simulink library "cjt_library_controllers"  (Simulink 9.0)
settings: Solver=ode45  StartTime=0.0  StopTime=10.0  RelTol=1e-3  EnableMultiTasking=on
values from neighbouring files (symbols this model uses):
  N = this.jointModel.n    [dataSheetGenerator.m]
undefined symbols (not defined in the file or in its folder): Cc, D, DiscIntNeverNeededParam, dob_switch, jointObj, K_lqr, kest
undefined symbols (not defined in the file): My_joint
libraries: cstblocks x6, cjt_library_observers x2
settings Model: Creator=wesley  LastModifiedBy=J�rn

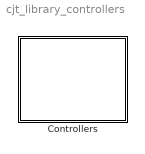
== system cjt_library_controllers ==
  Controllers : Subsystem

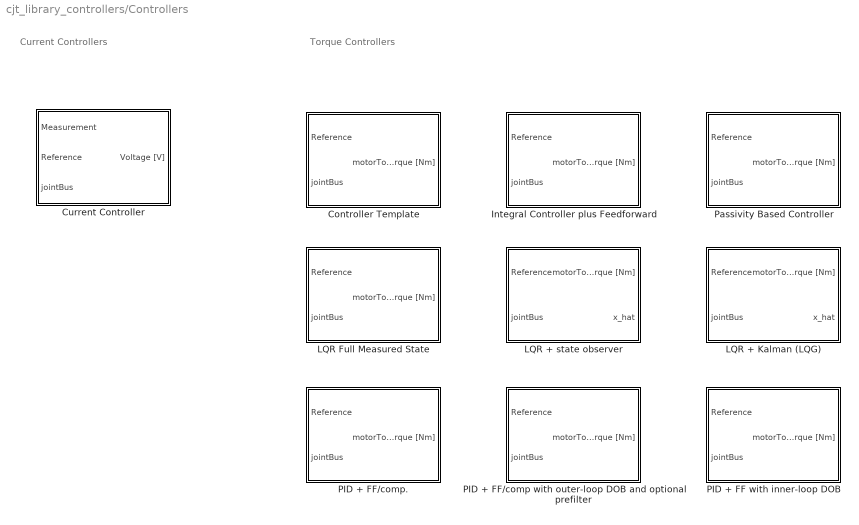
== system cjt_library_controllers/Controllers ==
  note: Torque Controllers
  note: Current Controllers
  Controller Template : Subsystem  mask(CJT Controller Template){jointObj=jointObj}
      mask prompts: jointObj "Joint Object"
      mask help:
      | This is a template block. If you have a controller that you wish to contribute to this library, this block here  represents your interface.
      |
      | Here are the steps to contribute your controller using this template:
      |
      | 1. Copy this block into your development. Disable and break its link to this library. You now have a copy of the interface in your model that is disconnected from the library.
      |
      | 2. Implement your controller within this block. The controller should use no hardcoded values. Wherever you can, access the properties of a CJT joint object. The joint object should be passed to the block through the mask as first parameter (e.g. jointObj).
      |
      | 3. Complete the block mask, so the user can specify all block properties programatically or manually through the mask.
      |
      | 4. Make an example:
      | a) Clean your development model up and convert it into a minimum example that demonstrates the use of your block.
      | b) Create an m-script that configures the required joint object and simulation parameters, runs the model.and displays some results. See existing examples and copy their format.
      | c) Write the documentation of your block.
      |
      | 5. Write a unit test. Look into the unit test directory and open the unit test file for this library. Add a test for your block. A good point to start is your example. Make the test pass.
      |
      | 6. Submit your contribution!
      |
      | Thanks a lot!
      |
      | 7.
      mask init:
      | % Do all the controller related computations here.
      | % Compute gains etc.
      | 
      | % E.g. get linear dynamics matrices first...
      | [A, B, C, I, D, K] = jointObj.getDynamicsMatrices();
      | 
      | % YOUR CODE HERE
      mask Help:
      | This is a template block. If you have a controller that you wish to contribute to this library, this block here  represents your interface.
      | 
      | Here are the steps to contribute your controller using this template:
      | 
      | 1. Copy this block into your development. Disable and break its link to this library. You now have a copy of the interface in your model that is disconnected from the library.
      | 
      | 2. Implement your controller within this block. The controller should use no hardcoded values. Wherever you can, access the properties of a CJT joint object. The joint object should be passed to the block through the mask as first parameter (e.g. jointObj).
      | 
      | 3. Complete the block mask, so the user can specify all block properties programatically or manually through the mask.
      | 
      | 4. Make an example:
      | a) Clean your development model up and convert it into a minimum example that demonstrates the use of your block.
      | b) Create an m-script that configures the required joint object and simulation parameters, runs the model.and displays some results. See existing examples and copy their format.
      | c) Write the documentation of your block.
      | 
      | 5. Write a unit test. Look into the unit test directory and open the unit test file for this library. Add a test for your block. A good point to start is your example. Make the test pass.
      | 
      | 6. Submit your contribution!
      | 
      | Thanks a lot!
  Current Controller : Subsystem  mask(CJT Torque Controller){jointObj=My_joint, P_Gain=1, I_Gain=0.05, ff_chk=on, bemf_chk=on}
      mask prompts: jointObj "Joint Object"; P_Gain "Proportional Gain"; I_Gain "Integral Gain"; ff_chk "Feedforward Action"; bemf_chk "Back EMF Compensation"
      mask help:
      | The block implements a PI current controller augmented by a voltage feedforward term and a back-EMF compensation based on motor velocity readings.
      |
      | This block serves in combination with an electrical subsystem block.
      |
      | Click >Help< for details on the parameters.
      mask init:
      | ff_enable = 0;
      | if ff_chk
      |     ff_enable = 1.0;
      | end
      | 
      | bemf_enable = 0;
      | if bemf_chk
      |     bemf_enable = 1.0;
      | end
      mask Help:
      | The block implements a PI current controller augmented by a voltage feedforward term and a back-EMF compensation based on motor velocity readings.
      | 
      | This block serves in combination with an electrical subsystem block.
      | 
      | <b>Mask parameters:</b>
      | 
      | Joint Object:  The class name of the CJT joint class name or the variable representing an instance of a CJT joint class, describing the
      | 
      | Proportional Gain: PI controller P-gain
      | Integral Gain: PI controller I-gain
      | 
      | Feedforward Action: check, if feedforward action is desired.
      | Back EMF Compensation : check, if back EMF compensation shall be active .
  Integral Controller plus Feedforward : Subsystem  mask(CJT Torque Controller){jointObj=jointObj, I_Gain=10}
      mask prompts: jointObj "Joint Object"; I_Gain "Integral gain K_I"
      mask help:
      | The block implements a torque controller comprised of a feedforward term complemented by an integral action with gain K_I to compensate for disturbances.
      |
      | Click >Help< for further documentation.
      mask Help:
      | The block implements a torque controller comprised of a feedforward term complemented by an integral action to compensate for disturbances. This type of controller has been used and discussed as lag-type control design in comparison to a pure feedforward action as well as a Proportional-Derivative control action in [1].
      | 
      | <b>Mask parameters:</b>
      | 
      | Joint Object:  The class name of the CJT joint class name or the variable representing an instance of a CJT joint class, describing the
      | 
      | K<sub>I</sub>: Integral gain
      | 
      | According to [1] the controller reduces disturbances up to a frequency <i>f = K<sub>I</sub>  / ( 2 PI ). </i>
      | 
      | <b>References:</b>
      | [1] D. Vischer and O. Khatib, â€œDesign and development of high-performance torque-controlled joints,â€ Robotics and Automation, IEEE Transactions on, vol. 11, no. 4, pp. 537â€“544, 1995.
      | [2] M. C. Readman, Flexible Joint Robots. CRC press, 1994.
  LQR + Kalman (LQG) : Subsystem  mask{jointObj=jointObj, outputIdx=7, Q=diag([0 0 1000 0 0 0]), R=5e-6, var_u=0.12^2, var_y=1.8e-10}
      mask prompts: jointObj "Joint Object (fixed output model)"; outputIdx "Measured output"; Q "State weighing matrix Q"; R "Input weighing matrix R"; var_u "Input noise variance"; var_y "Measurement noise variance"
      mask init:
      | % Get linear dynamics matrices
      | [A, B, C, D] = jointObj.getDynamicsMatrices();
      | 
      | % Parameters
      | N_outputs       = size(C,1);
      | 
      | % Get LQR gain and Kalman observer
      | [K_lqr, N]  	= getLQR(jointObj, outputIdx, Q, R);
      | [kest, L, Cc]	= getKalman(jointObj, outputIdx, var_u, var_y);
      | 
      | % Indexes of output states
      | kest_stateIdx   = kest.OutputGroup.StateEstimate;
      | 
      | % Discretize using Tustin transform
      | kest_tust       = c2d(kest, jointObj.Ts, 'tustin');
  LQR + state observer : Subsystem  mask{jointObj=jointObj, outputIdx=7, Q=diag([0 0 1000 0 0 0]), R=5e-6, place_gain=4}
      mask prompts: jointObj "Joint Object"; outputIdx "Measured output"; Q "State weighing matrix Q"; R "Input weighing matrix R"; place_gain "Pole placement gain"
      mask init:
      | % Get linear dynamics matrices
      | [A, B, C, D] = jointObj.getDynamicsMatrices();
      | 
      | % Parameters
      | N_outputs = size(C,1);
      | 
      | % Get LQR gain and state observer
      | [K_lqr, N]          = getLQR(jointObj, outputIdx, Q, R);
      | [sys_hat, L, Cc]	= getObserver(jointObj, outputIdx, place_gain, Q, R);
      | 
      | % Discretize using Tustin transform
      | sys_hat_tust = c2d(sys_hat, jointObj.Ts, 'tustin');
  LQR Full Measured State : Subsystem  mask{jointObj=My_joint, outputIdx=7, Q=diag([0 0 1000 0 0 0]), R=5e-6}
      mask prompts: jointObj "Joint Object"; outputIdx "Measured output"; Q "State weighing matrix Q"; R "Input weighing matrix R"
      mask init:
      | % Get linear dynamics matrices
      | [A, B, C, D] = jointObj.getDynamicsMatrices();
      | 
      | % Get LQR gain and premultiplication matrix N
      | [K_lqr, N]          = getLQR(jointObj, outputIdx, Q, R);
      | 
      | % Get selector to obtain full state from outputs y
      | % This makes use of the fact that the first 6 outputs are the states
      | outputToStates      = C(1:6,:)';
  PID + FF with inner-loop DOB : Subsystem  mask(PID + FF with inner-loop DOB){jointObj=jointObj, Kp=1, Ki=0, Kd=0, N=2*pi*200, ff_comp_switch=Feed-forward, DOB_enabled=on, f_c=100, measIdx=[7]}
      mask prompts: jointObj "Joint Object"; Kp "Proportional gain Kp"; Ki "Integral gain Ki"; Kd "Derivative gain Kd"; N "Filter coefficient N"; ff_comp_switch "Spring force rejection"; DOB_enabled "DOB enabled"; f_c "DOB cut-off frequency [Hz]"; measIdx "Measurement index"
      mask help:
      | This block implements a PID torque controller with optional feed-forward or compensation term, supplemented with an inner-loop DOB.
      |
      | Click >Help< for further documentation.
      mask init:
      | % Get linear dynamics matrices
      | [A, B, C, D, I, R, K] = jointObj.getDynamicsMatrices();
      mask Help:
      | This block implements a PID torque controller with optional feed-forward or compensation term, supplemented with an inner-loop DOB. The DOB is based on the nominal open-loop plant dynamics.
      | 
      | <b>Mask parameters:</b>
      | 
      | Joint Object: The class name of the CJT joint class name or the variable representing an instance of a CJT joint class.
      | K<sub>P</sub>, K<sub>I</sub>, K<sub>D</sub>: Proportional, derivative, and integral gain, respectively.
      | N: Derivative low-pass filter coefficient
      | DOB cutoff frequency: Cut-off frequency computed for the low-pass filter that must be used to make the inverse transfer function realisible.
      | Measurement index: Measured plant output that should be used for the DOB.
      | 
      | 
      | <b>References:</b>
      | 
      | H. S. Lee and M. Tomizuka, "Robust motion controller design for high-accuracy positioning systems". In IEEE Transactions on Industrial Electronics, vol. 43, no. 1, pp. 48--55, 1996.
      | 
      | W. Roozing, J. Malzahn, D. G. Caldwell, and N. G. Tsagarakis, "Comparison of open-loop and closed-loop disturbance observers for series elastic actuators". In Intelligent Robots and Systems (IROS), 2016 IEEE/RSJ International Conference on, 2016, pp. 3842--3847.
      | 
      | M. C. Readman, Flexible Joint Robots. CRC press, 1994.
      mask TypeOptions ff_comp_switch: Compensation | Feed-forward | Off
      mask Callback DOB_enabled:
      | % Toggle all DOB fields
      | fields = {  'f_c', ...
      |             'measIdx'
      |          };
      | toggleMaskFields(gcbh, 'DOB_enabled', fields, 'on');
      mask DialogControl Container3 Prompt: Controller
      mask DialogControl ParameterGroupVar Prompt: DOB parameters
  PID + FF/comp with outer-loop DOB and optional prefilter : Subsystem  mask(PID + FF/comp with outer-loop DOB and optional prefilter){jointObj=jointObj, Kp=0.1, Ki=0, Kd=0.001, N=2*pi*200, ff_comp_switch=Feed-forward, DOB_enable_switch=On, premult_enable_switch=Off, loadData=off, modelFname=DOB_results.mat, f_c_FF=50, f_c_DOB=80}
      mask prompts: jointObj "Joint Object"; Kp "Proportional gain Kp"; Ki "Integral gain Ki"; Kd "Derivative gain Kd"; N "Derivative filter coefficient N"; ff_comp_switch "Spring force rejection"; DOB_enable_switch "DOB"; premult_enable_switch "Premultiplication"; loadData "Load model/filters from file (see getLinearDOB_fromData)"; modelFname "Model/filters file (.mat)"; f_c_FF "Premultiplication (model inversion) cutoff frequency [Hz]"; f_c_DOB "DOB cutoff frequency [Hz]"
      mask help:
      | This block implements a PID torque controller with optional feed-forward or compensation term, supplemented with an outer-loop DOB and optional prefilter.
      |
      | Click >Help< for further documentation.
      mask init:
      | mask_PID_FFComp_OuterLoopDOB
      mask Help:
      | This block implements a PID torque controller with optional feed-forward or compensation term, supplemented with an outer-loop DOB and optional prefilter. The DOB is based on a nominal model of the closed control loop. Multiplication by the prefilter simply means taking the inverse of the closed-loop as premultiplication, with a low-pass filter, very similar to a classical lead filter.
      | 
      | <b>Mask parameters:</b>
      | 
      | Joint Object: The class name of the CJT joint class name or the variable representing an instance of a CJT joint class.
      | K<sub>P</sub>, K<sub>I</sub>, K<sub>D</sub>: Proportional, derivative, and integral gain, respectively.
      | N: Derivative low-pass filter coefficient
      | Models/filters file: Instead of analytical computation from the given joint model, a DOB model can be loaded from file, that is e.g. computed from experimental data.
      | Premultiplication and DOB cutoff frequency: Cut-off frequency computed for the low-pass filters that must be used to make the inverse transfer functions realisible.
      | 
      | 
      | <b>References:</b>
      | 
      | M. C. Readman, Flexible Joint Robots. CRC press, 1994.
      | 
      | K. Kong, J. Bae, and M. Tomizuka, "Control of Rotary Series Elastic Actuator for Ideal Force-Mode Actuation in Human-Robot Interaction Applications". In: IEEE/ASME Transactions on Mechatronics, vol. 14, no. 1, pp. 105--118, Feb. 2009.
      | 
      | N. Paine, S. Oh, and L. Sentis, "Design and Control Considerations for High-Performance Series Elastic Actuators". In: IEEE/ASME Transactions on Mechatronics, vol. 19, no. 3, pp. 1080--1091, Jun. 2014.
      | 
      | N. Paine, J. S. Mehling, J. Holley, N. A. Radford, G. Johnson, C.-L. Fok, and L. Sentis, "Actuator Control for the NASA-JSC Valkyrie Humanoid Robot: A Decoupled Dynamics Approach for Torque Control of Series Elastic Robots: Actuator Control for the NASA-JSC Valkyrie Humanoid Robot". In: Journal of Field Robotics, vol. 32, no. 3, pp. 378--396, May 2015.
      | 
      | J. S. Mehling, J. Holley, and M. K. O'Malley, "Leveraging disturbance observer based torque control for improved impedance rendering with series elastic actuators". In: IEEE/RSJ International Conference on Intelligent Robots and Systems (IROS), 2015, pp. 1646--1651.
      | 
      | W. Roozing, J. Malzahn, D. G. Caldwell, and N. G. Tsagarakis, "Comparison of open-loop and closed-loop disturbance observers for series elastic actuators". In:  IEEE/RSJ International Conference on Intelligent Robots and Systems (IROS), 2016, pp. 3842--3847.
      mask TypeOptions ff_comp_switch: Compensation | Feed-forward | Off
      mask TypeOptions DOB_enable_switch: Off | On
      mask Callback DOB_enable_switch:
      | % Toggle all DOB fields
      | fields = {  'premult_enable_switch', ...
      |             'loadData', ...
      |             'modelFname', ...
      |             'id_Np', ...
      |             'id_Nz', ...
      |             'f_c_FF', ...
      |             'f_c_DOB', ...
      |          };
      | toggleMaskFields(gcbh, 'DOB_enable_switch', fields, 'on');
      | 
      | % File load or model generation
      | if (strcmpi(get(gcbh, 'DOB_enable_switch'), 'on'))
      |     toggleMaskFields(gcbh, 'loadData', 'modelFname', 'on');
      |     toggleMaskFields(gcbh, 'loadData', {'f_c_FF', 'f_c_DOB'}, 'off');
      | end
      mask TypeOptions premult_enable_switch: Off | On
      mask Callback loadData:
      | if (strcmpi(get(gcbh, 'DOB_enable_switch'), 'on'))
      |     toggleMaskFields(gcbh, 'loadData', 'modelFname', 'on');
      |     toggleMaskFields(gcbh, 'loadData', {'button_build_DOB', 'f_c', 'id_Np', 'id_Nz', 'f_c_FF', 'f_c_DOB'}, 'off');
      | end
      mask DialogControl Container2 Prompt: Controller
      mask DialogControl DOB_container Prompt: DOB and premultiplication
      mask DialogControl DOB_analytical_container Prompt: Analytical DOB
  PID + FF/comp. : Subsystem  mask(PID + FF/comp.){jointObj=jointObj, Kp=2, Ki=0, Kd=0.01, N=2*pi*200, ff_comp_switch=Feed-forward}
      mask prompts: jointObj "Joint Object"; Kp "Proportional gain Kp"; Ki "Integral gain Ki"; Kd "Derivative gain Kd"; N "Filter coefficient N"; ff_comp_switch "Feed-forward/compensation"
      mask help:
      | This block implements a PID torque controller with optional feed-forward or compensation term.
      |
      | Click >Help< for further documentation.
      mask init:
      | % Get linear dynamics matrices
      | [A, B, C, D, I, R, K] = jointObj.getDynamicsMatrices();
      mask Help:
      | This block implements a PID torque controller with optional feed-forward or compensation term.
      | 
      | <b>Mask parameters:</b>
      | 
      | Joint Object: The class name of the CJT joint class name or the variable representing an instance of a CJT joint class.
      | K<sub>P</sub>, K<sub>I</sub>, K<sub>D</sub>: Proportional, derivative, and integral gain, respectively.
      | N: Derivative low-pass filter coefficient
      | 
      | 
      | <b>References:</b>
      | 
      | M. C. Readman, Flexible Joint Robots. CRC press, 1994.
      mask TypeOptions ff_comp_switch: Compensation | Feed-forward | Off
  Passivity Based Controller : Subsystem  mask(Passivity Based Torque Controller with Optional Generalized Momentum Based Disturbance Observer){jointObj=jointObj, BBinv=4, Ds=25, isDOBActive=on, L=2*pi*60}
      mask prompts: jointObj "Joint Object"; BBinv "Inertia Scaling"; Ds "Damping"; isDOBActive "DOB Active"; L "Gain L"
      mask help:
      | This block implements a passivity based torque controller. It has two positive valued parameters. The first parameter is a downscaling factor for the apparent inertia. The second parameter adds damping in proportion to the spring deflection rate. The controller relies on the knowledge of the joint intrinsic stiffness and damping provided through the joint class.
      |
      | The controller can be augmented by a generalized momentum based disturbance observer. The observer outputs a low-pass filtered version of the actual disturbance and  introduces one additional parameter. The parameter is the cut-off frequency of the low-pass filter in radians/s. The observer relies on the knowledge of the joint inertia provided through the joint class.
      |
      | Click >Help< for further documentation.
      mask init:
      | mask_Passivity_Based_Control
      mask Help:
      | This block implements the passivity based torque controller presented by Alin Albu-Schäffer, Christian Ott  and Gerd Hirzinger (2007).
      | It has two positive valued parameters. The first parameter is a downscaling factor for the apparent inertia. The second parameter adds damping in proportion to the spring deflection rate. The controller relies on the knowledge of the joint intrinsic stiffness and damping provided through the joint object.
      | 
      | The controller can be augmented by a generalized momentum based disturbance observer as described by Luc Le Tien  et al (2008).. The observer outputs a low-pass filtered version of the actual disturbance and  introduces one additional parameter. The parameter is the cut-off frequency of the low-pass filter in radians/s. The observer relies on the knowledge of the joint inertia provided through the joint class.
      | 
      | 
      | <b>Mask parameters:</b>
      | 
      | Joint Object: The class name of the CJT joint class name or the variable representing an instance of a CJT joint class.
      | Inertia Scaling: This parameter is a proportional gain on the torque error. It acts as an inertia downscaling factor. The apparent joint inertia proportionally increases for values < 0 and decreases for parameter values > 1
      | Damping: This parameter is a derivative gain on the joint deflection measurement. It adds damping in direct proportion to the joint deflection rate.
      | DOB Active: if checked, the controller is augmented by the generalized momentum based disturbance observer.
      | Gain L: Disturbance observer gain that essentially is the cut-off frequency of a low-pass filter for the actual real disturbance given in radians/s.
      | 
      | 
      | <b>References:</b>
      | Albu-Schäffer, Alin, Christian Ott, and Gerd Hirzinger. "A unified passivity-based control framework for position, torque and impedance control of flexible joint robots." The international journal of robotics research 26.1 (2007): 23-39.
      | 
      | Le Tien, Luc, et al. "Friction observer and compensation for control of robots with joint torque measurement." Intelligent Robots and Systems, 2008. IROS 2008. IEEE/RSJ International Conference on. IEEE, 2008.
      mask Callback isDOBActive:
      | maskObj = Simulink.Mask.get(gcb);
      | 
      | maskObj.Parameters(5).Enabled = maskObj.Parameters(4).Value;
      mask DialogControl Controller_container Prompt: Controller
      mask DialogControl DOB_container Prompt: Disturbance Observer (DOB)

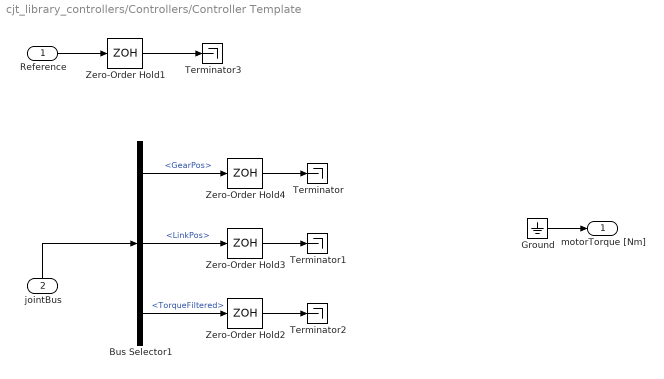
== system cjt_library_controllers/Controllers/Controller Template ==
  Reference : Inport
  jointBus : Inport  Port=2
  Bus Selector1 : BusSelector  OutputSignals=GearPos,LinkPos,TorqueFiltered
  Ground : Ground
  Terminator{,1..3} (4 alike) : Terminator
  Zero-Order Hold{1..4} (4 alike) : ZeroOrderHold  SampleTime=jointObj.Ts
  motorTorque [Nm] : Outport
  wires:
  jointBus/1 -> Bus Selector1/1
  Bus Selector1/1 -> Zero-Order Hold4/1  "<GearPos>"
  Bus Selector1/2 -> Zero-Order Hold3/1  "<LinkPos>"
  Bus Selector1/3 -> Zero-Order Hold2/1  "<TorqueFiltered>"
  Reference/1 -> Zero-Order Hold1/1
  Ground/1 -> motorTorque [Nm]/1
  Zero-Order Hold1/1 -> Terminator3/1
  Zero-Order Hold2/1 -> Terminator2/1
  Zero-Order Hold3/1 -> Terminator1/1
  Zero-Order Hold4/1 -> Terminator/1

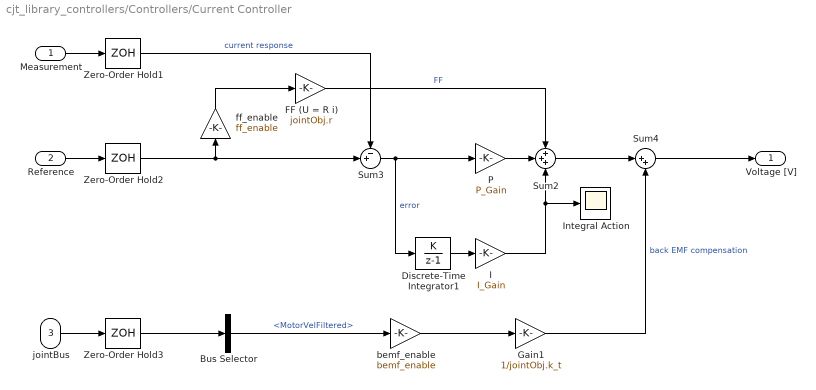
== system cjt_library_controllers/Controllers/Current Controller ==
  Measurement : Inport
  Reference : Inport  Port=2
  jointBus : Inport  Port=3
  Bus Selector : BusSelector  OutputSignals=MotorVelFiltered
  Discrete-Time Integrator1 : DiscreteIntegrator  IntegratorMethod=Accumulation: Forward Euler  SampleTime=jointObj.Ts_elec  ICPrevOutput=DiscIntNeverNeededParam  ICPrevScaledInput=DiscIntNeverNeededParam
  FF (U = R i) : Gain  Gain=jointObj.r
  Gain1 : Gain  Gain=1/jointObj.k_t
  I : Gain  Gain=I_Gain
  Integral Action : Scope
  P : Gain  Gain=P_Gain
  Sum2 : Sum  Inputs=+++
  Sum3 : Sum  Inputs=-+|
  Sum4 : Sum  Inputs=|++
  Zero-Order Hold1 : ZeroOrderHold  SampleTime=jointObj.Ts_elec
  Zero-Order Hold2 : ZeroOrderHold  SampleTime=jointObj.Ts_elec
  Zero-Order Hold3 : ZeroOrderHold  SampleTime=jointObj.Ts_elec
  bemf_enable : Gain  Gain=bemf_enable
  ff_enable : Gain  Gain=ff_enable
  Voltage [V] : Outport
  wires:
  Reference/1 -> Zero-Order Hold2/1
  jointBus/1 -> Zero-Order Hold3/1
  FF (U = R i)/1 -> Sum2/1  "FF"
  I/1 -> Sum2/3, Integral Action/1
  Discrete-Time Integrator1/1 -> I/1
  Sum2/1 -> Sum4/1
  Measurement/1 -> Zero-Order Hold1/1
  Gain1/1 -> Sum4/2  "back EMF compensation"
  P/1 -> Sum2/2
  Sum3/1 -> Discrete-Time Integrator1/1, P/1  "error"
  Bus Selector/1 -> bemf_enable/1  "<MotorVelFiltered>"
  ff_enable/1 -> FF (U = R i)/1
  bemf_enable/1 -> Gain1/1
  Zero-Order Hold1/1 -> Sum3/1  "current response"
  Zero-Order Hold2/1 -> ff_enable/1, Sum3/2
  Zero-Order Hold3/1 -> Bus Selector/1
  Sum4/1 -> Voltage [V]/1

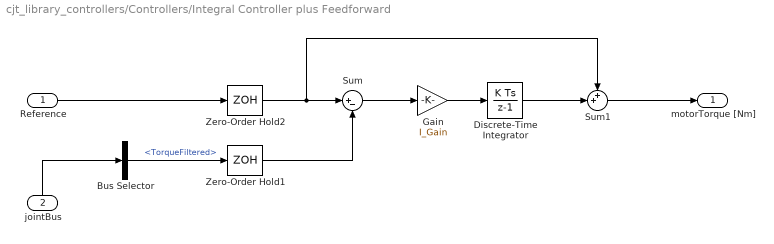
== system cjt_library_controllers/Controllers/Integral Controller plus Feedforward ==
  Reference : Inport
  jointBus : Inport  Port=2
  Bus Selector : BusSelector  OutputSignals=TorqueFiltered
  Discrete-Time Integrator : DiscreteIntegrator  InitialConditionSetting=State (most efficient)  SampleTime=jointObj.Ts  ICPrevOutput=DiscIntNeverNeededParam  ICPrevScaledInput=DiscIntNeverNeededParam
  Gain : Gain  Gain=I_Gain
  Sum : Sum  Inputs=|+-
  Sum1 : Sum  Inputs=++|
  Zero-Order Hold1 : ZeroOrderHold  SampleTime=jointObj.Ts
  Zero-Order Hold2 : ZeroOrderHold  SampleTime=jointObj.Ts
  motorTorque [Nm] : Outport
  wires:
  jointBus/1 -> Bus Selector/1
  Reference/1 -> Zero-Order Hold2/1
  Bus Selector/1 -> Zero-Order Hold1/1  "<TorqueFiltered>"
  Sum/1 -> Gain/1
  Gain/1 -> Discrete-Time Integrator/1
  Discrete-Time Integrator/1 -> Sum1/2
  Sum1/1 -> motorTorque [Nm]/1
  Zero-Order Hold1/1 -> Sum/2
  Zero-Order Hold2/1 -> Sum/1, Sum1/1

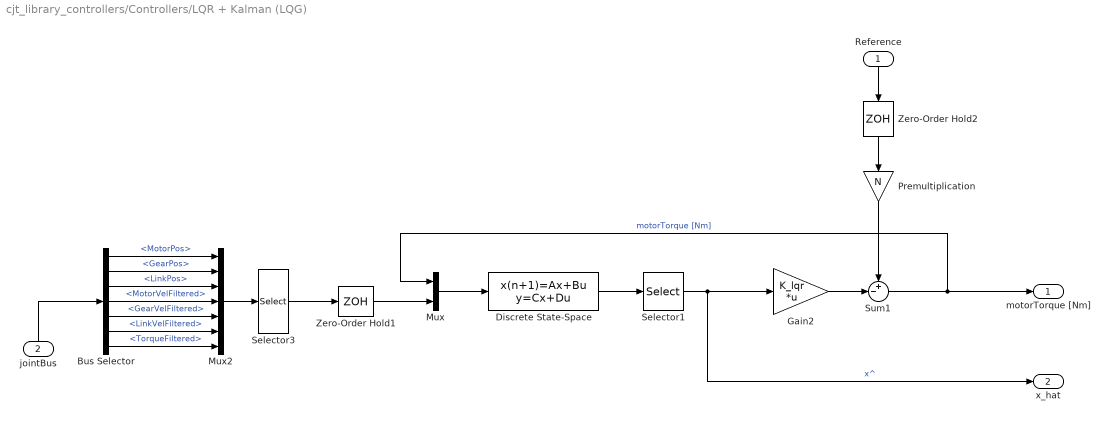
== system cjt_library_controllers/Controllers/LQR + Kalman (LQG) ==
  Reference : Inport
  jointBus : Inport  Port=2
  Bus Selector : BusSelector  OutputSignals=MotorPos,GearPos,LinkPos,MotorVelFiltered,GearVelFiltered,LinkVelFiltered,TorqueFiltered
  Discrete State-Space : DiscreteStateSpace  A=kest_tust.a  B=kest_tust.b  C=kest_tust.c  D=kest_tust.d  SampleTime=jointObj.Ts
  Gain2 : Gain  Gain=K_lqr  Multiplication=Matrix(K*u)
  Mux : Mux  Inputs=2
  Mux2 : Mux  Inputs=7
  Premultiplication : Gain  Gain=N
  Selector1 : Selector  InputPortWidth=size(kest.c,1)  IndexOptions=Index vector (dialog)  Indices=kest_stateIdx  OutputSizes=1
  Selector3 : Selector  InputPortWidth=N_outputs  IndexOptions=Index vector (dialog)  Indices=outputIdx  OutputSizes=1
  Sum1 : Sum  Inputs=+-|
  Zero-Order Hold1 : ZeroOrderHold  SampleTime=jointObj.Ts
  Zero-Order Hold2 : ZeroOrderHold  SampleTime=jointObj.Ts
  motorTorque [Nm] : Outport
  x_hat : Outport  Port=2
  wires:
  Discrete State-Space/1 -> Selector1/1
  Mux/1 -> Discrete State-Space/1
  Gain2/1 -> Sum1/2
  Premultiplication/1 -> Sum1/1
  Reference/1 -> Zero-Order Hold2/1
  Sum1/1 -> motorTorque [Nm]/1, Mux/1  "motorTorque [Nm]"
  Bus Selector/7 -> Mux2/7  "<TorqueFiltered>"
  Mux2/1 -> Selector3/1
  Bus Selector/1 -> Mux2/1  "<MotorPos>"
  Bus Selector/5 -> Mux2/5  "<GearVelFiltered>"
  Bus Selector/3 -> Mux2/3  "<LinkPos>"
  Bus Selector/6 -> Mux2/6  "<LinkVelFiltered>"
  Bus Selector/2 -> Mux2/2  "<GearPos>"
  Bus Selector/4 -> Mux2/4  "<MotorVelFiltered>"
  jointBus/1 -> Bus Selector/1
  Selector3/1 -> Zero-Order Hold1/1
  Selector1/1 -> x_hat/1, Gain2/1  "x^"
  Zero-Order Hold1/1 -> Mux/2
  Zero-Order Hold2/1 -> Premultiplication/1

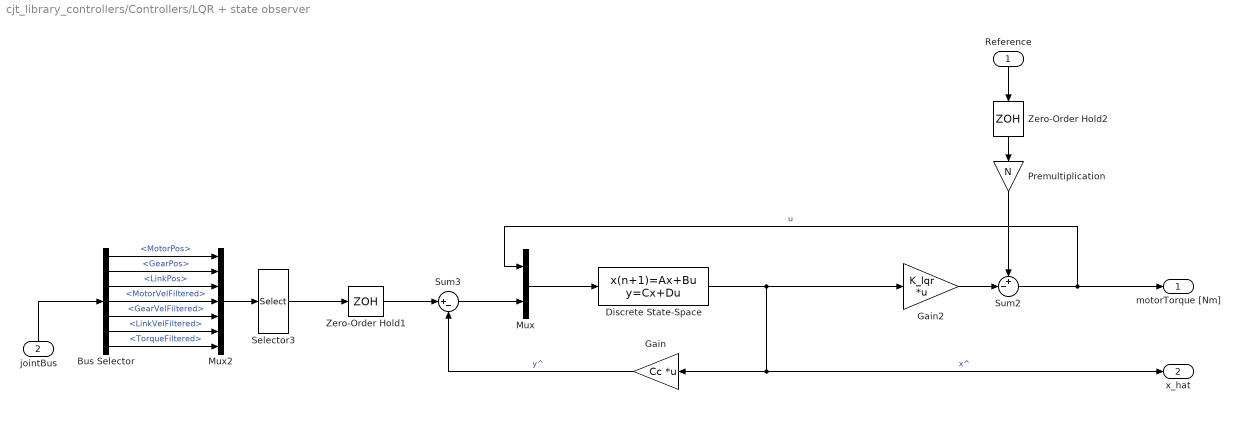
== system cjt_library_controllers/Controllers/LQR + state observer ==
  Reference : Inport
  jointBus : Inport  Port=2
  Bus Selector : BusSelector  OutputSignals=MotorPos,GearPos,LinkPos,MotorVelFiltered,GearVelFiltered,LinkVelFiltered,TorqueFiltered
  Discrete State-Space : DiscreteStateSpace  A=sys_hat_tust.a  B=sys_hat_tust.b  C=sys_hat_tust.c  D=sys_hat_tust.d  SampleTime=jointObj.Ts
  Gain : Gain  Gain=Cc  Multiplication=Matrix(K*u)
  Gain2 : Gain  Gain=K_lqr  Multiplication=Matrix(K*u)
  Mux : Mux  Inputs=2
  Mux2 : Mux  Inputs=7
  Premultiplication : Gain  Gain=N
  Selector3 : Selector  InputPortWidth=N_outputs  IndexOptions=Index vector (dialog)  Indices=outputIdx  OutputSizes=1
  Sum2 : Sum  Inputs=+-|
  Sum3 : Sum  Inputs=|+-
  Zero-Order Hold1 : ZeroOrderHold  SampleTime=jointObj.Ts
  Zero-Order Hold2 : ZeroOrderHold  SampleTime=jointObj.Ts
  motorTorque [Nm] : Outport
  x_hat : Outport  Port=2
  wires:
  Zero-Order Hold2/1 -> Premultiplication/1
  Zero-Order Hold1/1 -> Sum3/1
  Reference/1 -> Zero-Order Hold2/1
  Sum2/1 -> motorTorque [Nm]/1, Mux/1  "u"
  Premultiplication/1 -> Sum2/1
  Gain2/1 -> Sum2/2
  Mux/1 -> Discrete State-Space/1
  Selector3/1 -> Zero-Order Hold1/1
  Sum3/1 -> Mux/2
  Gain/1 -> Sum3/2  "y^"
  jointBus/1 -> Bus Selector/1
  Bus Selector/4 -> Mux2/4  "<MotorVelFiltered>"
  Bus Selector/2 -> Mux2/2  "<GearPos>"
  Bus Selector/6 -> Mux2/6  "<LinkVelFiltered>"
  Bus Selector/3 -> Mux2/3  "<LinkPos>"
  Bus Selector/5 -> Mux2/5  "<GearVelFiltered>"
  Bus Selector/1 -> Mux2/1  "<MotorPos>"
  Mux2/1 -> Selector3/1
  Discrete State-Space/1 -> x_hat/1, Gain/1, Gain2/1  "x^"
  Bus Selector/7 -> Mux2/7  "<TorqueFiltered>"

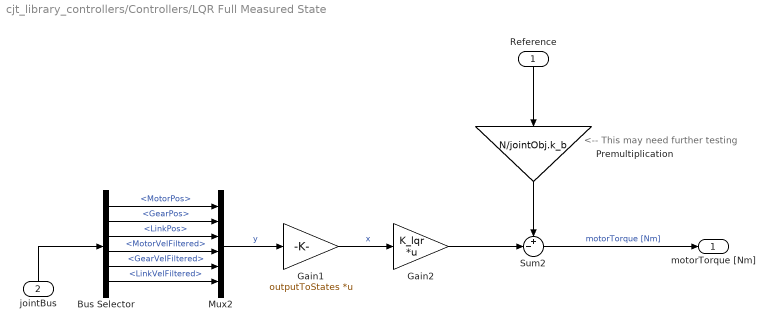
== system cjt_library_controllers/Controllers/LQR Full Measured State ==
  note: <-- This may need further testing
  Reference : Inport
  jointBus : Inport  Port=2
  Bus Selector : BusSelector  OutputSignals=MotorPos,GearPos,LinkPos,MotorVelFiltered,GearVelFiltered,LinkVelFiltered
  Gain1 : Gain  Gain=outputToStates  Multiplication=Matrix(K*u)
  Gain2 : Gain  Gain=K_lqr  Multiplication=Matrix(K*u)
  Mux2 : Mux  Inputs=6
  Premultiplication : Gain  Gain=N/jointObj.k_b
  Sum2 : Sum  Inputs=+-|
  motorTorque [Nm] : Outport
  wires:
  Gain1/1 -> Gain2/1  "x"
  Bus Selector/1 -> Mux2/1  "<MotorPos>"
  Bus Selector/5 -> Mux2/5  "<GearVelFiltered>"
  Bus Selector/3 -> Mux2/3  "<LinkPos>"
  Bus Selector/6 -> Mux2/6  "<LinkVelFiltered>"
  Bus Selector/2 -> Mux2/2  "<GearPos>"
  Bus Selector/4 -> Mux2/4  "<MotorVelFiltered>"
  jointBus/1 -> Bus Selector/1
  Gain2/1 -> Sum2/2
  Premultiplication/1 -> Sum2/1
  Sum2/1 -> motorTorque [Nm]/1  "motorTorque [Nm]"
  Reference/1 -> Premultiplication/1
  Mux2/1 -> Gain1/1  "y"

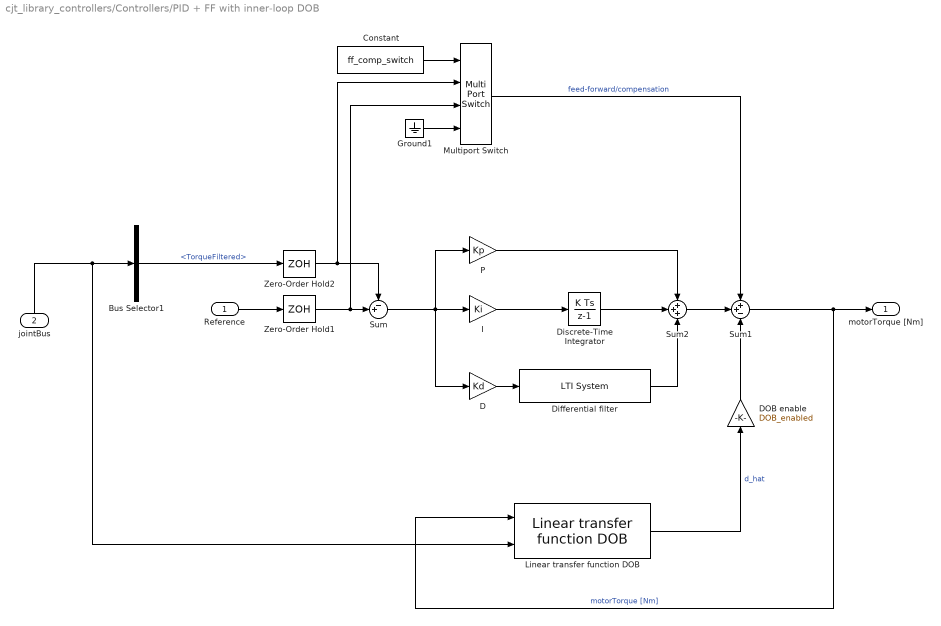
== system cjt_library_controllers/Controllers/PID + FF with inner-loop DOB ==
  Reference : Inport
  jointBus : Inport  Port=2
  Bus Selector1 : BusSelector  OutputSignals=TorqueFiltered
  Constant : Constant  Value=ff_comp_switch
  D : Gain  Gain=Kd
  DOB enable : Gain  Gain=DOB_enabled
  Differential filter : cstblocks/LTI System  sys=c2d(tf([N 0], [1, N]), jointObj.Ts, 'tustin')  IC=[]
  Discrete-Time Integrator : DiscreteIntegrator  SampleTime=-1  ICPrevOutput=DiscIntNeverNeededParam  ICPrevScaledInput=DiscIntNeverNeededParam
  Ground1 : Ground
  I : Gain  Gain=Ki
  Linear transfer function DOB : cjt_library_observers/Observers/Linear transfer function DOB  loadData=off  modelFname=DOB_results.mat  jointObj=jointObj  f_c=f_c  measIdx=measIdx  doPlot=off
  Multiport Switch : MultiPortSwitch
  P : Gain  Gain=Kp
  Sum : Sum  Inputs=-+|
  Sum1 : Sum  Inputs=++-
  Sum2 : Sum  Inputs=+++
  Zero-Order Hold1 : ZeroOrderHold  SampleTime=jointObj.Ts
  Zero-Order Hold2 : ZeroOrderHold  SampleTime=jointObj.Ts
  motorTorque [Nm] : Outport
  wires:
  Zero-Order Hold2/1 -> Sum/1, Multiport Switch/2
  Zero-Order Hold1/1 -> Sum/2, Multiport Switch/3
  Ground1/1 -> Multiport Switch/4
  Constant/1 -> Multiport Switch/1
  Multiport Switch/1 -> Sum1/1  "feed-forward/compensation"
  Reference/1 -> Zero-Order Hold1/1
  Sum1/1 -> Linear transfer function DOB/1, motorTorque [Nm]/1  "motorTorque [Nm]"
  Bus Selector1/1 -> Zero-Order Hold2/1  "<TorqueFiltered>"
  jointBus/1 -> Linear transfer function DOB/2, Bus Selector1/1
  Linear transfer function DOB/1 -> DOB enable/1  "d_hat"
  D/1 -> Differential filter/1
  I/1 -> Discrete-Time Integrator/1
  Discrete-Time Integrator/1 -> Sum2/2
  P/1 -> Sum2/1
  Differential filter/1 -> Sum2/3
  Sum2/1 -> Sum1/2
  Sum/1 -> D/1, I/1, P/1
  DOB enable/1 -> Sum1/3

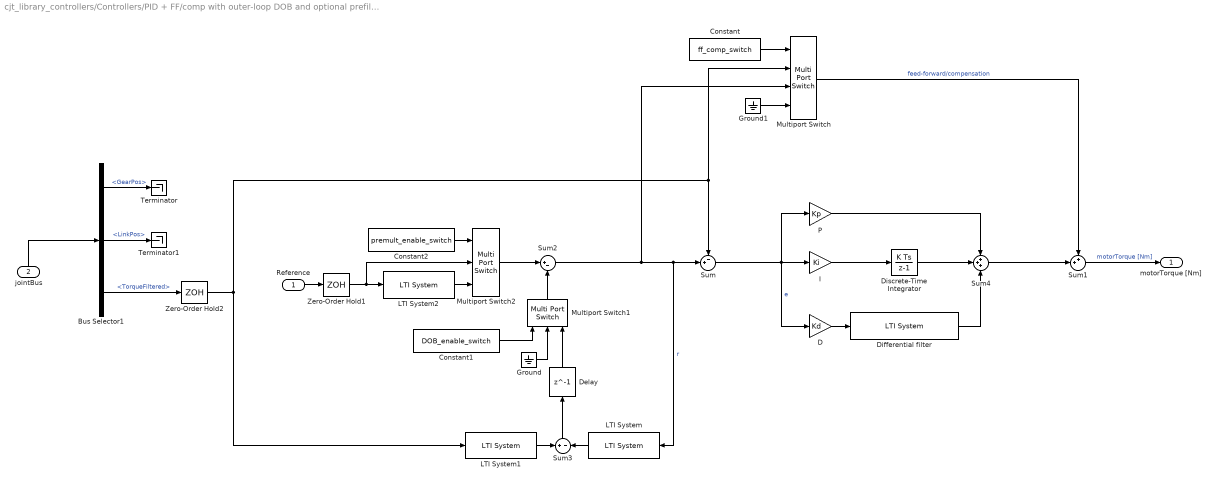
== system cjt_library_controllers/Controllers/PID + FF/comp with outer-loop DOB and optional prefilter ==
  Reference : Inport
  jointBus : Inport  Port=2
  Bus Selector1 : BusSelector  OutputSignals=GearPos,LinkPos,TorqueFiltered
  Constant : Constant  Value=ff_comp_switch
  Constant1 : Constant  Value=DOB_enable_switch
  Constant2 : Constant  Value=premult_enable_switch
  D : Gain  Gain=Kd
  Delay : Delay  DelayLength=1  InitialCondition=0
  Differential filter : cstblocks/LTI System  sys=c2d(tf([N 0], [1, N]), jointObj.Ts, 'tustin')  IC=[]
  Discrete-Time Integrator : DiscreteIntegrator  SampleTime=-1  ICPrevOutput=DiscIntNeverNeededParam  ICPrevScaledInput=DiscIntNeverNeededParam
  Ground : Ground
  Ground1 : Ground
  I : Gain  Gain=Ki
  LTI System : cstblocks/LTI System  sys=Q_td_d  IC=[]
  LTI System1 : cstblocks/LTI System  sys=PQ_td_d  IC=[]
  LTI System2 : cstblocks/LTI System  sys=PQ_ff_d  IC=[]
  Multiport Switch : MultiPortSwitch
  Multiport Switch1 : MultiPortSwitch  Inputs=2
  Multiport Switch2 : MultiPortSwitch  Inputs=2
  P : Gain  Gain=Kp
  Sum : Sum  Inputs=-+|
  Sum1 : Sum  Inputs=++|
  Sum2 : Sum  Inputs=|+-
  Sum3 : Sum  Inputs=+|-
  Sum4 : Sum  Inputs=+++
  Terminator : Terminator
  Terminator1 : Terminator
  Zero-Order Hold1 : ZeroOrderHold  SampleTime=jointObj.Ts
  Zero-Order Hold2 : ZeroOrderHold  SampleTime=jointObj.Ts
  motorTorque [Nm] : Outport
  wires:
  Delay/1 -> Multiport Switch1/3
  Multiport Switch2/1 -> Sum2/1
  Zero-Order Hold1/1 -> LTI System2/1, Multiport Switch2/2
  Zero-Order Hold2/1 -> LTI System1/1, Multiport Switch/2, Sum/1
  Reference/1 -> Zero-Order Hold1/1
  Ground1/1 -> Multiport Switch/4
  Bus Selector1/2 -> Terminator1/1  "<LinkPos>"
  Bus Selector1/1 -> Terminator/1  "<GearPos>"
  jointBus/1 -> Bus Selector1/1
  Bus Selector1/3 -> Zero-Order Hold2/1  "<TorqueFiltered>"
  Sum1/1 -> motorTorque [Nm]/1  "motorTorque [Nm]"
  Multiport Switch/1 -> Sum1/1  "feed-forward/compensation"
  Sum2/1 -> LTI System/1, Sum/2, Multiport Switch/3  "r"
  LTI System1/1 -> Sum3/1
  LTI System/1 -> Sum3/2
  Sum3/1 -> Delay/1
  LTI System2/1 -> Multiport Switch2/3
  Constant/1 -> Multiport Switch/1
  Multiport Switch1/1 -> Sum2/2
  Ground/1 -> Multiport Switch1/2
  Constant1/1 -> Multiport Switch1/1
  Constant2/1 -> Multiport Switch2/1
  D/1 -> Differential filter/1
  I/1 -> Discrete-Time Integrator/1
  Discrete-Time Integrator/1 -> Sum4/2
  P/1 -> Sum4/1
  Differential filter/1 -> Sum4/3
  Sum4/1 -> Sum1/2
  Sum/1 -> D/1, I/1, P/1  "e"

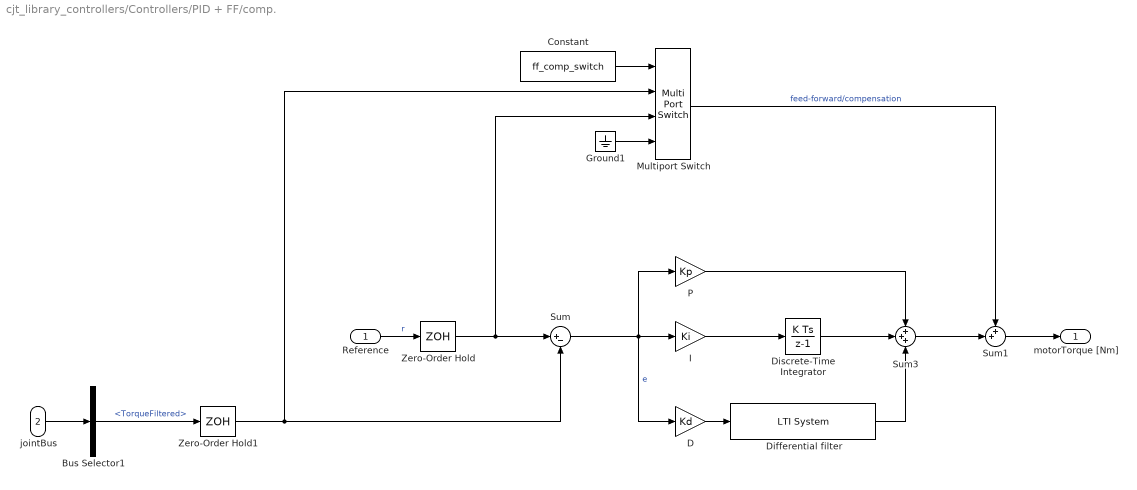
== system cjt_library_controllers/Controllers/PID + FF/comp. ==
  Reference : Inport
  jointBus : Inport  Port=2
  Bus Selector1 : BusSelector  OutputSignals=TorqueFiltered
  Constant : Constant  Value=ff_comp_switch
  D : Gain  Gain=Kd
  Differential filter : cstblocks/LTI System  sys=c2d(tf([N 0], [1, N]), jointObj.Ts, 'tustin')  IC=[]
  Discrete-Time Integrator : DiscreteIntegrator  SampleTime=-1  ICPrevOutput=DiscIntNeverNeededParam  ICPrevScaledInput=DiscIntNeverNeededParam
  Ground1 : Ground
  I : Gain  Gain=Ki
  Multiport Switch : MultiPortSwitch
  P : Gain  Gain=Kp
  Sum : Sum  Inputs=|+-
  Sum1 : Sum  Inputs=++|
  Sum3 : Sum  Inputs=+++
  Zero-Order Hold : ZeroOrderHold  SampleTime=jointObj.Ts
  Zero-Order Hold1 : ZeroOrderHold  SampleTime=jointObj.Ts
  motorTorque [Nm] : Outport
  wires:
  Zero-Order Hold1/1 -> Sum/2, Multiport Switch/2
  Zero-Order Hold/1 -> Multiport Switch/3, Sum/1
  Sum/1 -> P/1, I/1, D/1  "e"
  Sum3/1 -> Sum1/2
  Differential filter/1 -> Sum3/3
  P/1 -> Sum3/1
  Discrete-Time Integrator/1 -> Sum3/2
  I/1 -> Discrete-Time Integrator/1
  D/1 -> Differential filter/1
  Sum1/1 -> motorTorque [Nm]/1
  jointBus/1 -> Bus Selector1/1
  Ground1/1 -> Multiport Switch/4
  Bus Selector1/1 -> Zero-Order Hold1/1  "<TorqueFiltered>"
  Reference/1 -> Zero-Order Hold/1  "r"
  Constant/1 -> Multiport Switch/1
  Multiport Switch/1 -> Sum1/1  "feed-forward/compensation"

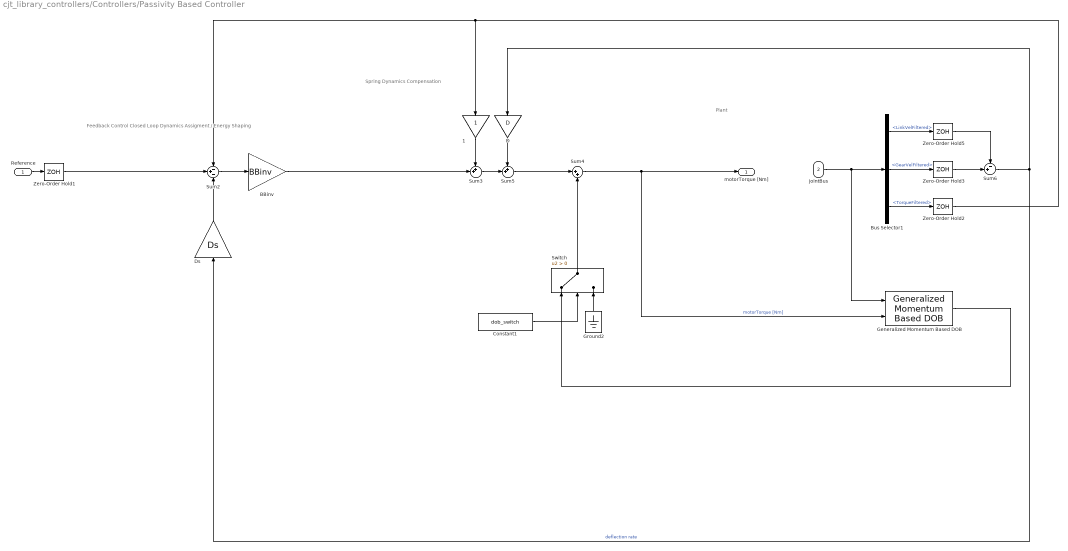
== system cjt_library_controllers/Controllers/Passivity Based Controller ==
  note: Feedback Control
      | Closed Loop Dynamics Assigment /
      | Energy Shaping
  note: Spring Dynamics Compensation
  note: Plant
  Reference : Inport
  jointBus : Inport  Port=2
  1 : Gain
  BBinv : Gain  Gain=BBinv
  Bus Selector1 : BusSelector  OutputSignals=LinkVelFiltered,GearVelFiltered,TorqueFiltered
  Constant1 : Constant  Value=dob_switch
  D : Gain  Gain=D
  Ds : Gain  Gain=Ds
  Generalized Momentum Based DOB : cjt_library_observers/Observers/Generalized Momentum Based DOB  jointObj=jointObj  L=L
  Ground2 : Ground
  Sum2 : Sum  Inputs=-+-
  Sum3 : Sum  Inputs=++|
  Sum4 : Sum  Inputs=|++
  Sum5 : Sum  Inputs=++|
  Sum6 : Sum  Inputs=-+|
  Switch : Switch  Criteria=u2 > Threshold
  Zero-Order Hold{1..3,5} (4 alike) : ZeroOrderHold  SampleTime=jointObj.Ts
  motorTorque [Nm] : Outport
  wires:
  Sum4/1 -> Generalized Momentum Based DOB/2, motorTorque [Nm]/1  "motorTorque [Nm]"
  jointBus/1 -> Generalized Momentum Based DOB/1, Bus Selector1/1
  Reference/1 -> Zero-Order Hold1/1
  Zero-Order Hold1/1 -> Sum2/2
  Bus Selector1/3 -> Zero-Order Hold2/1  "<TorqueFiltered>"
  Bus Selector1/2 -> Zero-Order Hold3/1  "<GearVelFiltered>"
  BBinv/1 -> Sum3/2
  Sum3/1 -> Sum5/2
  Sum5/1 -> Sum4/1
  Ground2/1 -> Switch/3
  Zero-Order Hold2/1 -> 1/1, Sum2/1
  Sum2/1 -> BBinv/1
  D/1 -> Sum5/1
  Sum6/1 -> Ds/1, D/1  "deflection rate"
  Bus Selector1/1 -> Zero-Order Hold5/1  "<LinkVelFiltered>"
  Zero-Order Hold5/1 -> Sum6/1
  Zero-Order Hold3/1 -> Sum6/2
  Ds/1 -> Sum2/3
  1/1 -> Sum3/1
  Switch/1 -> Sum4/2
  Generalized Momentum Based DOB/1 -> Switch/1
  Constant1/1 -> Switch/2
